simulink model "drone_control_tut3_R22a_2"  (R2022a)
settings: Solver=FixedStepAuto  StartTime=0.0  StopTime=inf  FixedStep=sample_time  RelTol=1e-3
PostLoadFcn:
  | load('drone_buses.mat');
model workspace (MAT data in the model file):
  SL_ROS_VariableLengthArrays_MaxSizes.CommonInfo.ArrayTruncateAction = 'EmitWarning'
  SL_ROS_VariableLengthArrays_MaxSizes.MsgTypeMap = containers.Map
  SL_ROS_VariableLengthArrays_MaxSizes.MsgTypeMap.serialization.keys = {'sensor_msgs/Image'}
  SL_ROS_VariableLengthArrays_MaxSizes.MsgTypeMap.serialization.values{1}(1).PropertyName = 'Data'
  SL_ROS_VariableLengthArrays_MaxSizes.MsgTypeMap.serialization.values{1}(1).DataType = 'uint8'
  SL_ROS_VariableLengthArrays_MaxSizes.MsgTypeMap.serialization.values{1}(1).MaxLength = 230400
  SL_ROS_VariableLengthArrays_MaxSizes.MsgTypeMap.serialization.values{1}(2).PropertyName = 'Encoding'
  SL_ROS_VariableLengthArrays_MaxSizes.MsgTypeMap.serialization.values{1}(2).DataType = 'uint8'
  SL_ROS_VariableLengthArrays_MaxSizes.MsgTypeMap.serialization.values{1}(2).MaxLength = 128
  SL_ROS_VariableLengthArrays_MaxSizes.MsgTypeMap.serialization.uniformity = 0
  SL_ROS_VariableLengthArrays_MaxSizes.MsgTypeMap.serialization.keyType = 'char'
  SL_ROS_VariableLengthArrays_MaxSizes.MsgTypeMap.serialization.valueType = 'any'
  cmd_calibration = 0.4
  sample_time = 0.05
undefined symbols (not defined in the file or in its folder): msg, Orientation, Position, publicar
libraries: robotlib x4, simulink_extras x2, simulink x2, aerolibanimutils x1
settings Model: Creator=rcasado  LastModifiedBy=usuario
settings SolverCC: AlgebraicLoopSolver=TrustRegion
settings DataIOCC: ReturnWorkspaceOutputs=off
settings OptimizationCC: EnhancedBackFolding=on  PassReuseOutputArgsAs=Individual arguments  ZeroExternalMemoryAtStartup=off  ZeroInternalMemoryAtStartup=off  MaxStackSize=64  OptimizeBlockOrder=speed  DifferentSizesBufferReuse=on  OptimizationCustomize=off  EfficientTunableParamExpr=on
settings DebuggingCC: ParameterTunabilityLossMsg=error  UnconnectedInputMsg=warning  UnconnectedOutputMsg=warning  UnconnectedLineMsg=warning  BusObjectLabelMismatch=none  PregeneratedLibrarySubsystemCodeDiagnostic=none  SFMachineParentedDataDiag=warning  ArithmeticOperatorsInVariantConditions=warning
settings HardwareCC: ProdBitPerPointer=32  ProdBitPerSizeT=32  ProdBitPerPtrDiffT=32  ProdLargestAtomicFloat=None  ProdIntDivRoundTo=Undefined  ProdEndianess=Unspecified  ProdWordSize=32  ProdHWDeviceType=Generic->Unspecified (assume 32-bit Generic)  UseEmbeddedCoderFeatures=off
settings SFSimCC: SimUseLocalCustomCode=off  MATLABDynamicMemAlloc=off  CustomCodeUndefinedFunction=UseInterfaceOnly
settings RTWCC: SystemTargetFile=ert.tlc  HardwareBoard=Robot Operating System (ROS)  TLCOptions="-aInlineSetEventsForThisBaseRateFcn=TLC_FALSE -aSuppressMultiTaskScheduler=TLC_FALSE  -aRateBasedStepFcn=0"  TemplateMakefile=ert_default_tmf  RTWUseLocalCustomCode=off  Toolchain=Catkin  TargetLang=C++  DLArmComputeVersion=19.05
settings CodeAppCC: ForceParamTrailComments=on  IgnoreCustomStorageClasses=off  OperatorAnnotations=on  SimulinkDataObjDesc=on  SFDataObjDesc=on  InsertBlockDesc=on
settings ERTTargetCC: SupportNonInlinedSFcns=on

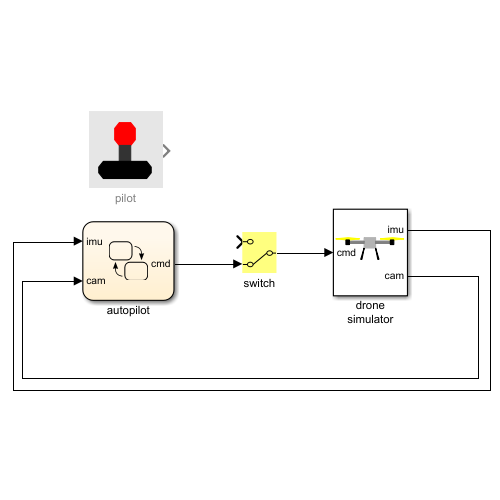
[thumbnail: Simulink's stored preview of the top-level diagram]
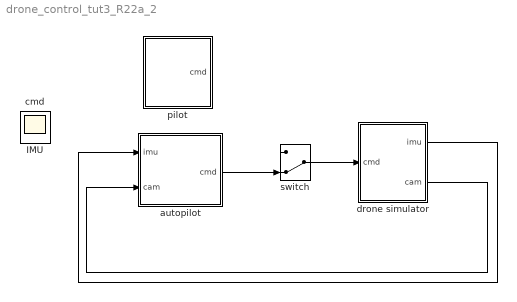
== system drone_control_tut3_R22a_2 ==
  autopilot : Stateflow chart  TreatAsAtomicUnit=on
  drone simulator : Subsystem
      mask Display:
      | patch([50 -50 -50 50], [40 40 -60 -60], [1 1 1])
      | 
      | patch([8 -8 -8 8], [6 6 -6 -6], [0.7 0.7 0.7])
      | 
      | patch([ 8  8  28  28], [2 0 0 2], [0.5 0.5 0.5])
      | patch([-8 -8 -28 -28], [2 0 0 2], [0.5 0.5 0.5])
      | 
      | patch([ 30  46  30  14], [6 5 4 5], [1 1 0])
      | patch([-30 -46 -30 -14], [6 5 4 5], [1 1 0])
      | 
      | patch([ 28  28  32  32], [4 -2 -2 4], [0 0 0])
      | patch([-28 -28 -32 -32], [4 -2 -2 4], [0 0 0])
      | 
      | patch([ 8  12  11  7], [-6 -18 -18 -6], [0 0 0])
      | patch([-8 -12 -11 -7], [-6 -18 -18 -6], [0 0 0])
  pilot : Subsystem
      mask Display:
      | patch([12 -2 -2 12], [12 12 -2 -2], [0.9 0.9 0.9])
      | 
      | % bola roja
      | patch([4 6 7 7 6 4 3 3], [6 6 7 9 10 10 9 7], [1 0 0])
      | 
      | % palo gris
      | patch([4 6 6 4], [3 3 6 6], [0.2 0.2 0.2])
      | 
      | % base negra
      | patch([1 9 10 10 9 1 0 0], [0 0 1 2 3 3 2 1], [0 0 0])
  switch : ManualSwitch  CurrentSetting=0
  IMU : Scope
  cmd : Scope
  wires:
  switch/1 -> drone simulator/1(cmd)
  autopilot/1(cmd) -> switch/2
  drone simulator/1(imu) -> autopilot/1(imu)
  drone simulator/2(cam) -> autopilot/2(cam)

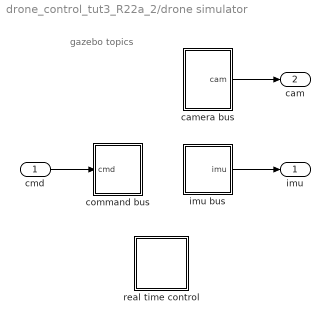
== system drone_control_tut3_R22a_2/drone simulator ==
  note: gazebo
      | topics
  cmd : Inport
  camera bus : Subsystem
  command bus : Subsystem
  imu bus : Subsystem
  real time control : Subsystem
      mask Display: disp('realtime\ncontrol')
  imu : Outport  VectorParamsAs1DForOutWhenUnconnected=off
  cam : Outport  Port=2  VectorParamsAs1DForOutWhenUnconnected=off
  wires:
  imu bus/1(imu) -> imu/1
  cmd/1 -> command bus/1(cmd)
  camera bus/1(cam) -> cam/1

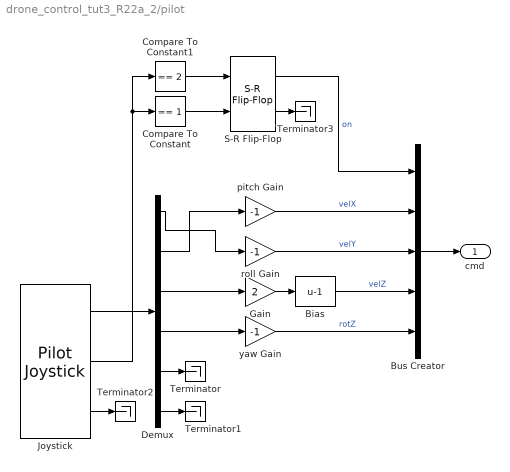
== system drone_control_tut3_R22a_2/pilot ==
  Bias : Bias  Bias=-1  SaturateOnIntegerOverflow=off
  Bus Creator : BusCreator  Inputs=5  OutDataTypeStr=Bus: bus_command  NonVirtualBus=on
      settings: InheritFromInputs=off
  Compare To Constant : simulink/Logic and Bit Operations/Compare To Constant  relop===  const=1  OutDataTypeStr=boolean
  Compare To Constant1 : simulink/Logic and Bit Operations/Compare To Constant  relop===  const=2  OutDataTypeStr=boolean
  Demux : Demux  Outputs=6
  Gain : Gain  Gain=2
  Joystick : aerolibanimutils/Pilot Joystick  JoystickID=Joystick1  OutputConfiguration=AllOutputs  SampleTime=sample_time
  S-R Flip-Flop : simulink_extras/Flip Flops/S-R Flip-Flop  initial_condition=0
  Terminator{,1..3} (4 alike) : Terminator
  pitch Gain : Gain  Gain=-1
  roll Gain : Gain  Gain=-1
  yaw Gain : Gain  Gain=-1
  cmd : Outport  VectorParamsAs1DForOutWhenUnconnected=off
  wires:
  Demux/4 -> yaw Gain/1
  Demux/3 -> Gain/1
  Demux/1 -> roll Gain/1
  Demux/2 -> pitch Gain/1
  Gain/1 -> Bias/1
  Bias/1 -> Bus Creator/4  "velZ"
  yaw Gain/1 -> Bus Creator/5  "rotZ"
  pitch Gain/1 -> Bus Creator/2  "velX"
  roll Gain/1 -> Bus Creator/3  "velY"
  S-R Flip-Flop/1 -> Bus Creator/1  "on"
  Bus Creator/1 -> cmd/1
  Joystick/1 -> Demux/1
  Demux/6 -> Terminator1/1
  Demux/5 -> Terminator/1
  Joystick/2 -> Compare To Constant1/1, Compare To Constant/1
  Joystick/3 -> Terminator2/1
  Compare To Constant/1 -> S-R Flip-Flop/2
  Compare To Constant1/1 -> S-R Flip-Flop/1
  S-R Flip-Flop/2 -> Terminator3/1

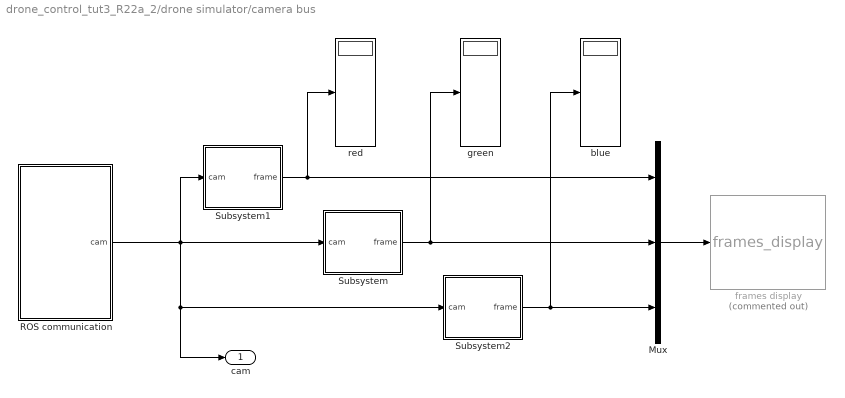
== system drone_control_tut3_R22a_2/drone simulator/camera bus ==
  Mux : Mux  Inputs=3
  ROS communication : Subsystem
  Subsystem : Subsystem
  Subsystem1 : Subsystem
  Subsystem2 : Subsystem
  blue : Display
  frames display : MATLABFcn  Commented=on  StartFcn=|  MATLABFcn=frames_display  OutputDimensions=0  Output1D=off
      | clear functions;
      | clc;
      mask Display:
      | patch([80 100 100 80], [60 60 80 80],[1 0 0])
      | 
      | patch([60 75 75 60], [20 20 30 30],[0 1 0])
      | 
      | patch([20 40 40 20], [40 40 50 50],[0 0 1])
  green : Display
  red : Display
  cam : Outport  VectorParamsAs1DForOutWhenUnconnected=off
  wires:
  Mux/1 -> frames display/1
  Subsystem/1(frame) -> green/1, Mux/2
  Subsystem2/1(frame) -> blue/1, Mux/3
  ROS communication/1(cam) -> cam/1, Subsystem2/1(cam), Subsystem1/1(cam), Subsystem/1(cam)
  Subsystem1/1(frame) -> red/1, Mux/1

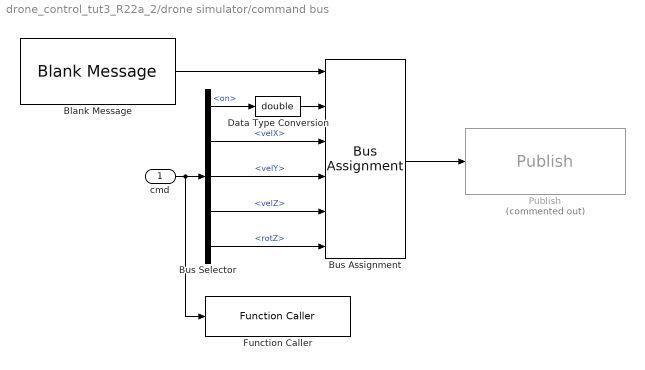
== system drone_control_tut3_R22a_2/drone simulator/command bus ==
  cmd : Inport
  Blank Message : robotlib/Blank Message  messageClass=Message  entityType=geometry_msgs/Pose  messageType=geometry_msgs/Pose  SampleTime=sample_time  legacyBusStruct=off
  Bus Assignment : BusAssignment  AssignedSignals=Position.X,Orientation.X,Orientation.Y,Orientation.Z,Orientation.W
  Bus Selector : BusSelector  OutputSignals=on,velX,velY,velZ,rotZ
  Data Type Conversion : DataTypeConversion  OutDataTypeStr=double  SaturateOnIntegerOverflow=off  RndMeth=Floor
  Function Caller : FunctionCaller  FunctionPrototype=publicar(msg)
  Publish : robotlib/Publish  Commented=on  topicSource=Select from ROS network  topic=/quadcopter2/bus_command  messageType=geometry_msgs/Pose  legacyBusStruct=off  messageQueueLength=105
  wires:
  Bus Assignment/1 -> Publish/1
  cmd/1 -> Function Caller/1, Bus Selector/1
  Blank Message/1 -> Bus Assignment/1
  Bus Selector/4 -> Bus Assignment/5  "<velZ>"
  Bus Selector/3 -> Bus Assignment/4  "<velY>"
  Bus Selector/2 -> Bus Assignment/3  "<velX>"
  Bus Selector/1 -> Data Type Conversion/1  "<on>"
  Bus Selector/5 -> Bus Assignment/6  "<rotZ>"
  Data Type Conversion/1 -> Bus Assignment/2
  ? -> ?

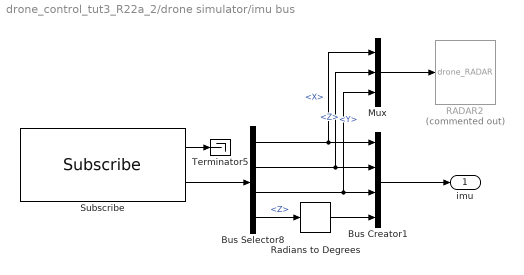
== system drone_control_tut3_R22a_2/drone simulator/imu bus ==
  Bus Creator1 : BusCreator  Inputs=4  OutDataTypeStr=Bus: bus_IMU  NonVirtualBus=on
      settings: InheritFromInputs=off
  Bus Selector8 : BusSelector  DialogController=Simulink.DDGSource_BusSelector  OutputSignals=Pose.Position.X,Pose.Position.Y,Pose.Position.Z,Pose.Orientation.Z
  Mux : Mux  Inputs=3
  RADAR2 : MATLABFcn  Commented=on  StartFcn=|  MATLABFcn=drone_RADAR  OutputDimensions=0  Output1D=off
      | clear functions;
      | clc;
      mask Display:
      | plot([00 10], [05 05])
      | plot([05 05], [00 10])
      | 
      | plot([01 09 09 01 01], [01 01 09 09 01])
      | plot([03 07 07 03 03], [03 03 07 07 03])
  Radians to Degrees : simulink_extras/Transformations/Radians to Degrees
  Subscribe : robotlib/Subscribe  topicSource=Select from ROS network  topic=/quadcopter2/odometry  messageType=gazebo_msgs/ModelState  SampleTime=sample_time  legacyBusStruct=off  messageQueueLength=51
  Terminator5 : Terminator
  imu : Outport  VectorParamsAs1DForOutWhenUnconnected=off
  wires:
  Subscribe/1 -> Terminator5/1
  Bus Selector8/4 -> Radians to Degrees/1  "<Z>"
  Bus Selector8/2 -> Bus Creator1/2, Mux/2  "<Y>"
  Bus Selector8/3 -> Bus Creator1/3, Mux/3  "<Z>"
  Bus Selector8/1 -> Bus Creator1/1, Mux/1  "<X>"
  Bus Creator1/1 -> imu/1
  Radians to Degrees/1 -> Bus Creator1/4
  Subscribe/2 -> Bus Selector8/1
  Mux/1 -> RADAR2/1

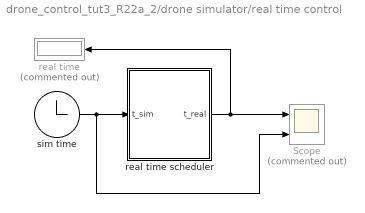
== system drone_control_tut3_R22a_2/drone simulator/real time control ==
  Scope : Scope  Commented=on  NumInputPorts=2
  real time : Display  Commented=on
      settings: Format=bank
  real time scheduler : MATLAB Function  TreatAsAtomicUnit=on
  sim time : Clock
  wires:
  real time scheduler/1(t_real) -> real time/1, Scope/1
  sim time/1 -> real time scheduler/1(t_sim), Scope/2

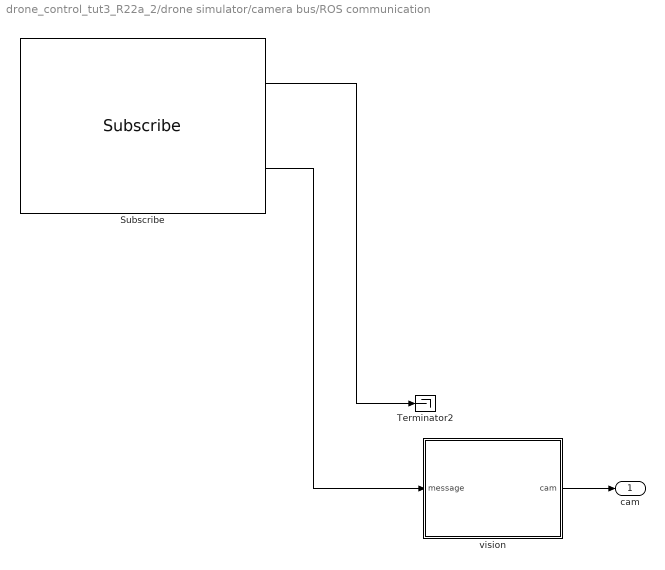
== system drone_control_tut3_R22a_2/drone simulator/camera bus/ROS communication ==
  Subscribe : robotlib/Subscribe  topicSource=Select from ROS network  topic=/quadcopter2/onboard_camera/image_raw  messageType=sensor_msgs/Image  SampleTime=sample_time  legacyBusStruct=off  messageQueueLength=51
  Terminator2 : Terminator
  vision : MATLAB Function  TreatAsAtomicUnit=on
  cam : Outport  VectorParamsAs1DForOutWhenUnconnected=off
  wires:
  vision/1(cam) -> cam/1
  Subscribe/2 -> vision/1(message)
  Subscribe/1 -> Terminator2/1

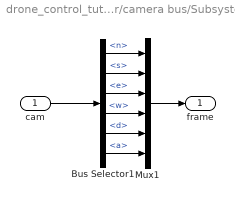
== system drone_control_tut3_R22a_2/drone simulator/camera bus/Subsystem ==
  cam : Inport
  Bus Selector1 : BusSelector  OutputSignals=green.n,green.s,green.e,green.w,green.d,green.a
  Mux1 : Mux  Inputs=6
  frame : Outport  VectorParamsAs1DForOutWhenUnconnected=off
  wires:
  Bus Selector1/3 -> Mux1/3  "<e>"
  Bus Selector1/6 -> Mux1/6  "<a>"
  Bus Selector1/5 -> Mux1/5  "<d>"
  Bus Selector1/4 -> Mux1/4  "<w>"
  cam/1 -> Bus Selector1/1
  Bus Selector1/1 -> Mux1/1  "<n>"
  Mux1/1 -> frame/1
  Bus Selector1/2 -> Mux1/2  "<s>"

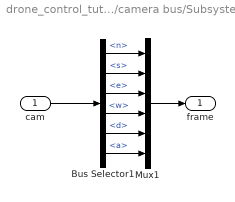
== system drone_control_tut3_R22a_2/drone simulator/camera bus/Subsystem1 ==
  cam : Inport
  Bus Selector1 : BusSelector  OutputSignals=red.n,red.s,red.e,red.w,red.d,red.a
  Mux1 : Mux  Inputs=6
  frame : Outport  VectorParamsAs1DForOutWhenUnconnected=off
  wires:
  Bus Selector1/3 -> Mux1/3  "<e>"
  Bus Selector1/6 -> Mux1/6  "<a>"
  Bus Selector1/5 -> Mux1/5  "<d>"
  Bus Selector1/4 -> Mux1/4  "<w>"
  cam/1 -> Bus Selector1/1
  Bus Selector1/1 -> Mux1/1  "<n>"
  Mux1/1 -> frame/1
  Bus Selector1/2 -> Mux1/2  "<s>"

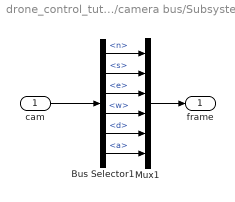
== system drone_control_tut3_R22a_2/drone simulator/camera bus/Subsystem2 ==
  cam : Inport
  Bus Selector1 : BusSelector  OutputSignals=blue.n,blue.s,blue.e,blue.w,blue.d,blue.a
  Mux1 : Mux  Inputs=6
  frame : Outport  VectorParamsAs1DForOutWhenUnconnected=off
  wires:
  Bus Selector1/3 -> Mux1/3  "<e>"
  Bus Selector1/6 -> Mux1/6  "<a>"
  Bus Selector1/5 -> Mux1/5  "<d>"
  Bus Selector1/4 -> Mux1/4  "<w>"
  cam/1 -> Bus Selector1/1
  Bus Selector1/1 -> Mux1/1  "<n>"
  Mux1/1 -> frame/1
  Bus Selector1/2 -> Mux1/2  "<s>"

== matlab function drone_control_tut3_R22a_2/drone simulator/camera bus/ROS communication/vision ==
  data: message input; cam output Bus: bus_camera
function cam = fcn(message)

% leemos la imagen
width  = message.Width;
height = message.Height;
img    = message.Data;

% establecemos los valores umbrales de deteccion de color
th1 = 50;         % umbral entre color primario y secundarios
th2 = 20;         % umbral entre colores secundarios

% marco rojo
frame_red.d = +inf;        % distancia estimada
frame_red.a = +inf;        % angulo de entrada estimado
frame_red.n = +inf;        % lado norte
frame_red.s = -inf;        % lado sur
frame_red.e = -inf;        % lado este
frame_red.w = +inf;        % lado oeste

% marco verde
frame_green = frame_red;      
% marco azul
frame_blue = frame_red; 


% deteccion de rectangulos conteniendo los pixeles de cada marco
i = 1;
for row = 1:height %240
for col = 1:width  %320

    r = double(img(i));  i=i+1;
    g = double(img(i));  i=i+1;
    b = double(img(i));  i=i+1;
    
    if(abs(g-b) < th2) && ((r-g) > th1)        %rojo
        if(frame_red.n > row) 
           frame_red.n = double(row);
        end
        if(frame_red.s < row) 
           frame_red.s = double(row);
        end
        if(frame_red.e < col) 
           frame_red.e = double(col);
        end
        if(frame_red.w > col) 
           frame_red.w = double(col);
        end
    elseif(abs(b-r) < th2) && ((g-b) > th1)    %verde
        if(frame_green.n > row) 
           frame_green.n = double(row);
        end
        if(frame_green.s < row) 
           frame_green.s = double(row);
        end
        if(frame_green.e < col) 
           frame_green.e = double(col);
        end
        if(frame_green.w > col) 
           frame_green.w = double(col);
        end
    elseif(abs(r-g) < th2) && ((b-r) > th1)    %azul
        if(frame_blue.n > row) 
           frame_blue.n = double(row);
        end
        if(frame_blue.s < row) 
           frame_blue.s = double(row);
        end
        if(frame_blue.e < col) 
           frame_blue.e = double(col);
        end
        if(frame_blue.w > col) 
           frame_blue.w = double(col);
        end
    end
    
end
end

% Cambio del sistema de coordenadas de la imagen
frame_red.n   = 120 - frame_red.n;
frame_red.s   = 120 - frame_red.s;
frame_red.e   = frame_red.e - 161;
frame_red.w   = frame_red.w - 161;

frame_green.n = 120 - frame_green.n;
frame_green.s = 120 - frame_green.s;
frame_green.e = frame_green.e - 161;
frame_green.w = frame_green.w - 161;

frame_blue.n  = 120 - frame_blue.n;
frame_blue.s  = 120 - frame_blue.s;
frame_blue.e  = frame_blue.e - 161;
frame_blue.w  = frame_blue.w - 161;


%% Analisis de posicion (distancia, y angulos de deriva/entrada)

d2 = 160^2;    % 160^2 pixeles
L  = 0.23;       % alto de marco
A  = 0.43;       % ancho del marco

if frame_red.n > -inf && frame_red.n < 119 && frame_red.s > -120
    l = frame_red.n - frame_red.s;
    h = frame_red.s + l/2;
    frame_red.d = L/l * sqrt(d2 + h^2);
    ap = frame_red.e - frame_red.w;
    a = max(A/L * l,ap);
    frame_red.a = acosd(ap/a);
end

if frame_green.n > -inf && frame_green.n < 119 && frame_green.s > -120
    l = frame_green.n - frame_green.s;
    h = frame_green.s + l/2;
    frame_green.d = L/l * sqrt(d2 + h^2);
    ap = frame_green.e - frame_green.w;
    a = max(A/L * l,ap);
    frame_green.a = acosd(ap/a);
end

if frame_blue.n > -inf && frame_blue.n < 119 && frame_blue.s > -120
    l = frame_blue.n - frame_blue.s;
    h = frame_blue.s + l/2;
    frame_blue.d = L/l * sqrt(d2 + h^2);
    ap = frame_blue.e - frame_blue.w;
    a = max(A/L * l,ap);
    frame_blue.a = acosd(ap/a);
end




%% Enviamos informacion por el topic
cam.red = frame_red;
cam.green = frame_green;
cam.blue = frame_blue;

== matlab function drone_control_tut3_R22a_2/drone simulator/real time control/real time scheduler ==
  data: t_sim input; t_real output
function t_real = fcn(t_sim)
%#codegen

coder.extrinsic('tic');
coder.extrinsic('toc');

persistent t0;
if isempty(t0)
    t0 = tic;
    t_real = 0;
end

t_real = toc(t0);

t_dif = t_sim - t_real;
if t_dif > 0
%    disp(t_dif)
    pause(t_dif);
end

t_real = toc(t0);
%disp(t_real)

== stateflow chart drone_control_tut3_R22a_2/autopilot ==
  settings: updateMethod=DISCRETE  sampleTime=sample_time  executeAtInitialization=1
  state RedFrame
    state Go2Center
      entry:
    state FrameVisible
      entry:
      Hover();
      during:
      Look2Frame('red');
      cmd.velX = min((cam.red.d-0.4)/2,1);
    state Turning
      entry:
      Hover();
      cmd.rotZ = 1;
    state FrameClose
      entry:
      Hover
      initA = cam.red.a
    state ShiftLeft
      entry:
      cmd.velY = 0.1;
      during:
      Look2Frame('red');
      cmd.velX = (cam.red.d-0.3)/8;
    state ShiftRight
      entry:
      cmd.velY = -0.1;
      during:
      Look2Frame('red');
      cmd.velX = (cam.red.d-0.3)/8;
    state Crossing
      entry:
      Hover
      cmd.velX = 0.3;
      during:
      Look2Frame('red');
    state GoingUp
      entry:
      Hover
      cmd.velZ = 0.3;
    state End
    (default) -> RedFrame.Go2Center
    RedFrame.Go2Center -> RedFrame.FrameVisible [order 1] : [cam.red.d ~= inf]
    RedFrame.FrameVisible -> RedFrame.Go2Center [order 2] : [cam.red.d == inf]
    RedFrame.Go2Center -> RedFrame.Turning [order 2] : [Fly2(0, 0, 2)<0.2]
    RedFrame.Turning -> RedFrame.FrameVisible : [cam.red.d ~= inf]
    RedFrame.FrameVisible -> RedFrame.FrameClose [order 1] : [cam.red.d < 0.45]
    RedFrame.FrameClose -> RedFrame.ShiftLeft
    RedFrame.ShiftLeft -> RedFrame.ShiftRight [order 2] : [initA < cam.red.a]
    RedFrame.ShiftRight -> RedFrame.Crossing : [cam.red.a < 3]
    RedFrame.ShiftLeft -> RedFrame.Crossing [order 1] : [cam.red.a < 3]
    RedFrame.Crossing -> RedFrame.GoingUp : [after(4,sec)]
    RedFrame.GoingUp -> RedFrame.End : [after(2,sec)]
  state GreenFrame
    state Go2Center
      entry:
    state FrameVisible
      entry:
      Hover();
      during:
      Look2Frame('green');
      cmd.velX = min((cam.green.d-0.4)/2,1);
    state Turning
      entry:
      Hover();
      cmd.rotZ = 1;
      cmd.velZ = -0.2;
    state FrameClose
      entry:
      Hover
      initA = cam.green.a
    state ShiftLeft
      entry:
      cmd.velY = 0.1;
      during:
      Look2Frame('green');
      cmd.velX = (cam.green.d-0.3)/8;
    state ShiftRight
      entry:
      cmd.velY = -0.1;
      during:
      Look2Frame('green');
      cmd.velX = (cam.green.d-0.3)/8;
    state Crossing
      entry:
      Hover
      cmd.velX = 0.3;
      during:
      Look2Frame('green');
    state GoingUp
      entry:
      Hover
      cmd.velZ = 0.3;
    state End
    (default) -> GreenFrame.Go2Center
    GreenFrame.Go2Center -> GreenFrame.FrameVisible [order 1] : [cam.green.d ~= inf]
    GreenFrame.FrameVisible -> GreenFrame.Go2Center [order 2] : [cam.green.d == inf]
    GreenFrame.Go2Center -> GreenFrame.Turning [order 2] : [Fly2(0, 0, 2)<0.2]
    GreenFrame.Turning -> GreenFrame.FrameVisible : [cam.green.d ~= inf]
    GreenFrame.FrameVisible -> GreenFrame.FrameClose [order 1] : [cam.green.d < 0.45]
    GreenFrame.FrameClose -> GreenFrame.ShiftLeft
    GreenFrame.ShiftLeft -> GreenFrame.ShiftRight [order 2] : [initA < cam.green.a]
    GreenFrame.ShiftRight -> GreenFrame.Crossing : [cam.green.a < 3]
    GreenFrame.ShiftLeft -> GreenFrame.Crossing [order 1] : [cam.green.a < 3]
    GreenFrame.Crossing -> GreenFrame.GoingUp : [after(4,sec)]
    GreenFrame.GoingUp -> GreenFrame.End : [after(2,sec)]
  state BlueFrame
    state Go2Center
      entry:
    state FrameVisible
      entry:
      Hover();
      during:
      Look2Frame('blue');
      cmd.velX = min((cam.blue.d-0.4)/2,1);
    state Turning
      entry:
      Hover();
      cmd.rotZ = 1;
    state FrameClose
      entry:
      Hover
      initA = cam.blue.a
    state ShiftLeft
      entry:
      cmd.velY = 0.1;
      during:
      Look2Frame('blue');
      cmd.velX = (cam.blue.d-0.3)/8;
    state ShiftRight
      entry:
      cmd.velY = -0.1;
      during:
      Look2Frame('blue');
      cmd.velX = (cam.blue.d-0.3)/8;
    state Crossing
      entry:
      Hover
      cmd.velX = 0.3;
      during:
      Look2Frame('blue');
    state GoingUp
      entry:
      Hover
      cmd.velZ = 0.3;
    state End
    (default) -> BlueFrame.Go2Center
    BlueFrame.Go2Center -> BlueFrame.FrameVisible [order 1] : [cam.blue.d ~= inf]
    BlueFrame.FrameVisible -> BlueFrame.Go2Center [order 2] : [cam.blue.d == inf]
    BlueFrame.Go2Center -> BlueFrame.Turning [order 2] : [Fly2(0, 0, 2)<0.2]
    BlueFrame.Turning -> BlueFrame.FrameVisible : [cam.blue.d ~= inf]
    BlueFrame.FrameVisible -> BlueFrame.FrameClose [order 1] : [cam.blue.d < 0.45]
    BlueFrame.FrameClose -> BlueFrame.ShiftLeft
    BlueFrame.ShiftLeft -> BlueFrame.ShiftRight [order 2] : [initA < cam.blue.a]
    BlueFrame.ShiftRight -> BlueFrame.Crossing : [cam.blue.a < 3]
    BlueFrame.ShiftLeft -> BlueFrame.Crossing [order 1] : [cam.blue.a < 3]
    BlueFrame.Crossing -> BlueFrame.GoingUp : [after(4,sec)]
    BlueFrame.GoingUp -> BlueFrame.End : [after(2,sec)]
  state TakeOff
    state End
    state SetBase
      entry:
      posXinit = imu.posX;
      posYinit = imu.posY;
      posZinit = imu.posZ;
    state Start
      entry:
      Hover();
    SetBase -> TakeOff.End : [Fly2(posXinit, posYinit, 1)<0.1]
    Start -> SetBase
    (default) -> Start
  state Landing
    state Go2Base
    state Stop
      entry:
      cmd.on = false;
    (default) -> Go2Base
    Go2Base -> Stop : [Fly2(posXinit, posYinit, 0.6)<0.05]
  TakeOff.End -> RedFrame
  (default) -> TakeOff
  RedFrame.End -> GreenFrame
  GreenFrame.End -> BlueFrame
  BlueFrame.End -> Landing
  data: X function_input; d3D function_output; Y function_input; Z function_input; id function_input; imu input Bus: bus_IMU size=1; cmd output Bus: bus_command size=1; cam input Bus: bus_camera size=1; posZinit local; posYinit local; posXinit local; initA local
  function d3D = Fly2(X,Y,Z):
    | function d3D = Fly2(X,Y,Z)
    | 
    | % target distance decomposed into earth axes
    | dxe = X - imu.posX;
    | dye = Y - imu.posY;
    | dze = Z - imu.posZ;
    | 
    | % target distance
    | d3D = norm([dxe;dye;dze]);
    | 
    | % target distance on the plane
    | d2D = norm([dxe;dye]);
    | 
    | % angle between drone heading and target
    | bearing = atan2d(dye, dxe) - imu.rumbo;
    | 
    | % target distance decomposed into drone body axes
    | dx = d2D * cosd(bearing);
    | dy = d2D * sind(bearing);
    | dz = dze;
    | 
    | % velocity obtained from distance
    | vel = [dx;dy;dz]/2;
    | if norm(vel) > 1 
    |     vel = vel / norm(vel);
    | end
    | 
    | cmd.velX = vel(1);
    | cmd.velY = vel(2);
    | cmd.velZ = vel(3);
  function Hover:
    | function Hover
    | 
    | cmd.on   = true;
    | cmd.velX = 0;
    | cmd.velY = 0;
    | cmd.velZ = 0;
    | cmd.rotZ = 0;
  function Look2Frame(id):
    | function Look2Frame(id)
    | 
    | switch id
    |     case 'red'
    |         fr = cam.red;
    |     case 'green'
    |         fr = cam.green;
    |     case 'blue'
    |         fr = cam.blue;
    | end
    | 
    | if (fr.d ~= inf)
    |     HorCenter = (fr.e + fr.w)/2;
    |     cmd.rotZ  = - HorCenter/80;
    |     VerCenter = (fr.n + fr.s)/2;
    |     cmd.velZ  = VerCenter/120;
    | end
